simulink model "signal_generating"  (R2019b)
settings: Solver=VariableStepAuto  StartTime=0.0  StopTime=2  MaxStep=0.1e-3  RelTol=1e-3
settings Model: Creator=raobo  LastModifiedBy=raobo

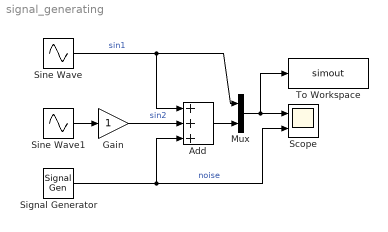
== system signal_generating ==
  Add : Sum  Inputs=+++
  Gain : Gain
  Mux : Mux  Inputs=2
  Scope : Scope  NumInputPorts=2
  Signal Generator : SignalGenerator  WaveForm=random  Amplitude=0.1  Units=rad/sec
  Sine Wave : Sin  Frequency=200  SampleTime=0
  Sine Wave1 : Sin  Frequency=2*pi*50  SampleTime=0
  To Workspace : ToWorkspace  VariableName=simout  SaveFormat=Timeseries  SampleTime=-1
  wires:
  Sine Wave1/1 -> Gain/1
  Mux/1 -> To Workspace/1, Scope/1
  Add/1 -> Mux/2
  Gain/1 -> Add/2  "sin2"
  Sine Wave/1 -> Add/1, Mux/1  "sin1"
  Signal Generator/1 -> Scope/2, Add/3  "noise"
